simulink model "two_axes_motor_control"  (R2018a)
settings: Solver=VariableStepAuto  StartTime=0.0  StopTime=2700  RelTol=1e-3
undefined symbols (not defined in the file): b, J, Km, La, max_current, max_speed, Ra
libraries: simulink x6
settings Model: Creator=Ivonne  LastModifiedBy=Ivonne

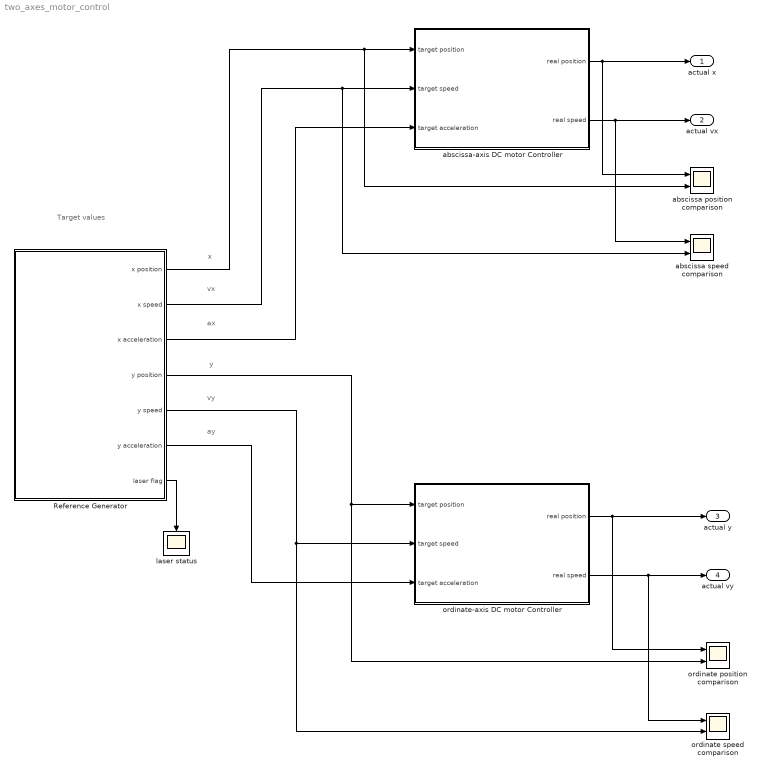
== system two_axes_motor_control ==
  note: x
  note: Target values
  note: vx
  note: ax
  note: y
  note: vy
  note: ay
  "Reference Generator " : Subsystem
  abscissa position comparison : Scope  NumInputPorts=2
  abscissa speed comparison : Scope  NumInputPorts=2
  abscissa-axis DC motor Controller : Subsystem
  laser status : Scope
  ordinate position comparison : Scope  NumInputPorts=2
  ordinate speed comparison : Scope  NumInputPorts=2
  ordinate-axis DC motor Controller : Subsystem
  actual x : Outport
  actual vx : Outport  Port=2
  actual y : Outport  Port=3
  actual vy : Outport  Port=4
  wires:
  "Reference Generator "/1("x position ") -> abscissa position comparison/2, abscissa-axis DC motor Controller/1(target position)
  "Reference Generator "/3("x acceleration ") -> abscissa-axis DC motor Controller/3(target acceleration)
  "Reference Generator "/2("x speed ") -> abscissa speed comparison/2, abscissa-axis DC motor Controller/2(target speed)
  "Reference Generator "/7("laser flag ") -> laser status/1
  abscissa-axis DC motor Controller/1(real position) -> abscissa position comparison/1, actual x/1
  abscissa-axis DC motor Controller/2(real speed) -> abscissa speed comparison/1, actual vx/1
  "Reference Generator "/4("y position ") -> ordinate position comparison/2, ordinate-axis DC motor Controller/1(target position)
  ordinate-axis DC motor Controller/1(real position) -> actual y/1, ordinate position comparison/1
  "Reference Generator "/6("y acceleration ") -> ordinate-axis DC motor Controller/3(target acceleration)
  "Reference Generator "/5("y speed ") -> ordinate-axis DC motor Controller/2(target speed), ordinate speed comparison/2
  ordinate-axis DC motor Controller/2(real speed) -> ordinate speed comparison/1, actual vy/1

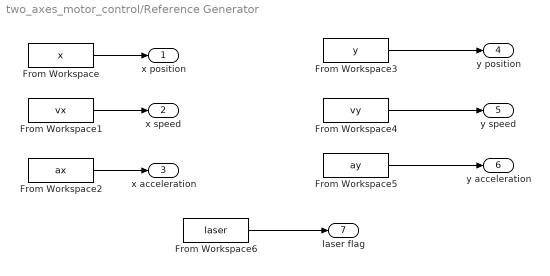
== system two_axes_motor_control/Reference Generator  ==
  From Workspace : FromWorkspace  VariableName=x  SampleTime=0  OutputAfterFinalValue=Holding final value
  From Workspace1 : FromWorkspace  VariableName=vx  SampleTime=0  OutputAfterFinalValue=Holding final value
  From Workspace2 : FromWorkspace  VariableName=ax  SampleTime=0  OutputAfterFinalValue=Holding final value
  From Workspace3 : FromWorkspace  VariableName=y  SampleTime=0  OutputAfterFinalValue=Holding final value
  From Workspace4 : FromWorkspace  VariableName=vy  SampleTime=0  OutputAfterFinalValue=Holding final value
  From Workspace5 : FromWorkspace  VariableName=ay  SampleTime=0  OutputAfterFinalValue=Holding final value
  From Workspace6 : FromWorkspace  VariableName=laser  SampleTime=0  Interpolate=off  OutputAfterFinalValue=Setting to zero
  "x position " : Outport
  "x speed " : Outport  Port=2
  "x acceleration " : Outport  Port=3
  "y position " : Outport  Port=4
  "y speed " : Outport  Port=5
  "y acceleration " : Outport  Port=6
  "laser flag " : Outport  Port=7
  wires:
  From Workspace/1 -> "x position "/1
  From Workspace5/1 -> "y acceleration "/1
  From Workspace3/1 -> "y position "/1
  From Workspace6/1 -> "laser flag "/1
  From Workspace2/1 -> "x acceleration "/1
  From Workspace4/1 -> "y speed "/1
  From Workspace1/1 -> "x speed "/1

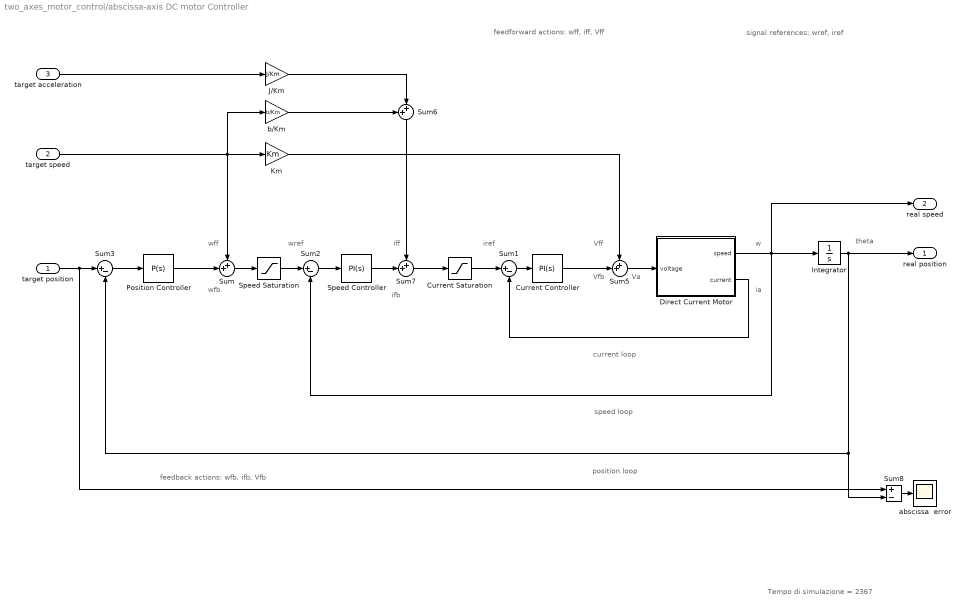
== system two_axes_motor_control/abscissa-axis DC motor Controller ==
  note: Tempo di simulazione = 2367
  note: ia
  note: theta
  note: w
  note: Va
  note: Vfb
  note: Vff
  note: signal references: wref, iref
  note: iref
  note: ifb
  note: iff
  note: wref
  note: wfb
  note: wff
  note: feedforward actions: wff, iff, Vff
  note: position loop
  note: speed loop
  note: current loop
  note: feedback actions: wfb, ifb, Vfb
  target position : Inport
  target speed : Inport  Port=2
  target acceleration : Inport  Port=3
  Current Controller : simulink/Continuous/PID Controller  Controller=PI  TimeDomain=Continuous-time  SampleTime=-1  IntegratorMethod=Forward Euler  FilterMethod=Forward Euler  Form=Parallel  UseFilter=on  ControllerParametersSource=internal  P=5000  I=10000  D=0  N=100  InitialConditionSource=internal  InitialConditionForIntegrator=0  InitialConditionForFilter=0  ExternalReset=none  LimitOutput=off  UpperSaturationLimit=inf  LowerSaturationLimit=-inf  LinearizeAsGain=on  AntiWindupMode=none  Kb=1  TrackingMode=off  Kt=1  PParamMin=[]  PParamMax=[]  IParamMin=[]  IParamMax=[]  DParamMin=[]  DParamMax=[]  NParamMin=[]  NParamMax=[]  KbParamMin=[]  KbParamMax=[]  KtParamMin=[]  KtParamMax=[]  POutMin=[]  POutMax=[]  IOutMin=[]  IOutMax=[]  DOutMin=[]  DOutMax=[]  NOutMin=[]  NOutMax=[]  KbOutMin=[]  KbOutMax=[]  KtOutMin=[]  KtOutMax=[]  IntegratorOutMin=[]  IntegratorOutMax=[]  FilterOutMin=[]  FilterOutMax=[]  SumOutMin=[]  SumOutMax=[]  SumI1OutMin=[]  SumI1OutMax=[]  SumI2OutMin=[]  SumI2OutMax=[]  SumI3OutMin=[]  SumI3OutMax=[]  SumDOutMin=[]  SumDOutMax=[]  SaturationOutMin=[]  SaturationOutMax=[]  IntegratorContinuousStateAttributes=''  IntegratorStateMustResolveToSignalObject=off  IntegratorRTWStateStorageClass=Auto  FilterContinuousStateAttributes=''  FilterStateMustResolveToSignalObject=off  FilterRTWStateStorageClass=Auto  DifferentiatorICPrevScaledInput=0  DifferentiatorOutMin=[]  DifferentiatorOutMax=[]  FilterDiffOutCoefMin=[]  FilterDiffOutCoefMax=[]  SumDenOutMin=[]  SumDenOutMax=[]  SumNumOutMin=[]  SumNumOutMax=[]  ReciprocalOutMin=[]  ReciprocalOutMax=[]  DivideOutMin=[]  DivideOutMax=[]  TunerSelectOption=Frequency Response Based
  Current Saturation : Saturate  UpperLimit=max_current  LowerLimit=-max_current
  Direct Current Motor : Subsystem
  Integrator : Integrator
  J/Km : Gain  Gain=J/Km
  Km : Gain  Gain=Km
  Position Controller : simulink/Continuous/PID Controller  Controller=P  TimeDomain=Continuous-time  SampleTime=-1  IntegratorMethod=Forward Euler  FilterMethod=Forward Euler  Form=Parallel  UseFilter=on  ControllerParametersSource=internal  P=10  I=1  D=0  N=100  InitialConditionSource=internal  InitialConditionForIntegrator=0  InitialConditionForFilter=0  ExternalReset=none  LimitOutput=off  UpperSaturationLimit=inf  LowerSaturationLimit=-inf  LinearizeAsGain=on  AntiWindupMode=none  Kb=1  TrackingMode=off  Kt=1  PParamMin=[]  PParamMax=[]  IParamMin=[]  IParamMax=[]  DParamMin=[]  DParamMax=[]  NParamMin=[]  NParamMax=[]  KbParamMin=[]  KbParamMax=[]  KtParamMin=[]  KtParamMax=[]  POutMin=[]  POutMax=[]  IOutMin=[]  IOutMax=[]  DOutMin=[]  DOutMax=[]  NOutMin=[]  NOutMax=[]  KbOutMin=[]  KbOutMax=[]  KtOutMin=[]  KtOutMax=[]  IntegratorOutMin=[]  IntegratorOutMax=[]  FilterOutMin=[]  FilterOutMax=[]  SumOutMin=[]  SumOutMax=[]  SumI1OutMin=[]  SumI1OutMax=[]  SumI2OutMin=[]  SumI2OutMax=[]  SumI3OutMin=[]  SumI3OutMax=[]  SumDOutMin=[]  SumDOutMax=[]  SaturationOutMin=[]  SaturationOutMax=[]  IntegratorContinuousStateAttributes=''  IntegratorStateMustResolveToSignalObject=off  IntegratorRTWStateStorageClass=Auto  FilterContinuousStateAttributes=''  FilterStateMustResolveToSignalObject=off  FilterRTWStateStorageClass=Auto  DifferentiatorICPrevScaledInput=0  DifferentiatorOutMin=[]  DifferentiatorOutMax=[]  FilterDiffOutCoefMin=[]  FilterDiffOutCoefMax=[]  SumDenOutMin=[]  SumDenOutMax=[]  SumNumOutMin=[]  SumNumOutMax=[]  ReciprocalOutMin=[]  ReciprocalOutMax=[]  DivideOutMin=[]  DivideOutMax=[]  TunerSelectOption=Frequency Response Based
  Speed Controller : simulink/Continuous/PID Controller  Controller=PI  TimeDomain=Continuous-time  SampleTime=-1  IntegratorMethod=Forward Euler  FilterMethod=Forward Euler  Form=Parallel  UseFilter=on  ControllerParametersSource=internal  P=200  I=400  D=0  N=100  InitialConditionSource=internal  InitialConditionForIntegrator=0  InitialConditionForFilter=0  ExternalReset=none  LimitOutput=off  UpperSaturationLimit=inf  LowerSaturationLimit=-inf  LinearizeAsGain=on  AntiWindupMode=none  Kb=1  TrackingMode=off  Kt=1  PParamMin=[]  PParamMax=[]  IParamMin=[]  IParamMax=[]  DParamMin=[]  DParamMax=[]  NParamMin=[]  NParamMax=[]  KbParamMin=[]  KbParamMax=[]  KtParamMin=[]  KtParamMax=[]  POutMin=[]  POutMax=[]  IOutMin=[]  IOutMax=[]  DOutMin=[]  DOutMax=[]  NOutMin=[]  NOutMax=[]  KbOutMin=[]  KbOutMax=[]  KtOutMin=[]  KtOutMax=[]  IntegratorOutMin=[]  IntegratorOutMax=[]  FilterOutMin=[]  FilterOutMax=[]  SumOutMin=[]  SumOutMax=[]  SumI1OutMin=[]  SumI1OutMax=[]  SumI2OutMin=[]  SumI2OutMax=[]  SumI3OutMin=[]  SumI3OutMax=[]  SumDOutMin=[]  SumDOutMax=[]  SaturationOutMin=[]  SaturationOutMax=[]  IntegratorContinuousStateAttributes=''  IntegratorStateMustResolveToSignalObject=off  IntegratorRTWStateStorageClass=Auto  FilterContinuousStateAttributes=''  FilterStateMustResolveToSignalObject=off  FilterRTWStateStorageClass=Auto  DifferentiatorICPrevScaledInput=0  DifferentiatorOutMin=[]  DifferentiatorOutMax=[]  FilterDiffOutCoefMin=[]  FilterDiffOutCoefMax=[]  SumDenOutMin=[]  SumDenOutMax=[]  SumNumOutMin=[]  SumNumOutMax=[]  ReciprocalOutMin=[]  ReciprocalOutMax=[]  DivideOutMin=[]  DivideOutMax=[]  TunerSelectOption=Frequency Response Based
  Speed Saturation : Saturate  UpperLimit=max_speed  LowerLimit=-max_speed
  Sum{,5..7} (4 alike) : Sum  Inputs=++|
  Sum1 : Sum  Inputs=|+-
  Sum2 : Sum  Inputs=|+-
  Sum3 : Sum  Inputs=|+-
  Sum8 : Sum  Inputs=+-
  abscissa  error : Scope
  b/Km : Gain  Gain=b/Km
  real position : Outport
  real speed : Outport  Port=2
  wires:
  Sum6/1 -> Sum7/1
  Direct Current Motor/1(speed) -> Sum2/2, Integrator/1, real speed/1
  Current Saturation/1 -> Sum1/1
  target speed/1 -> b/Km/1, Km/1, Sum/1
  Sum2/1 -> Speed Controller/1
  Speed Saturation/1 -> Sum2/1
  target position/1 -> Sum8/1, Sum3/1
  Current Controller/1 -> Sum5/2
  Sum5/1 -> Direct Current Motor/1(voltage)
  b/Km/1 -> Sum6/1
  Speed Controller/1 -> Sum7/2
  Position Controller/1 -> Sum/2
  Integrator/1 -> Sum8/2, Sum3/2, real position/1
  target acceleration/1 -> J/Km/1
  Direct Current Motor/2(current) -> Sum1/2
  Sum3/1 -> Position Controller/1
  Sum/1 -> Speed Saturation/1
  J/Km/1 -> Sum6/2
  Km/1 -> Sum5/1
  Sum1/1 -> Current Controller/1
  Sum7/1 -> Current Saturation/1
  Sum8/1 -> abscissa  error/1

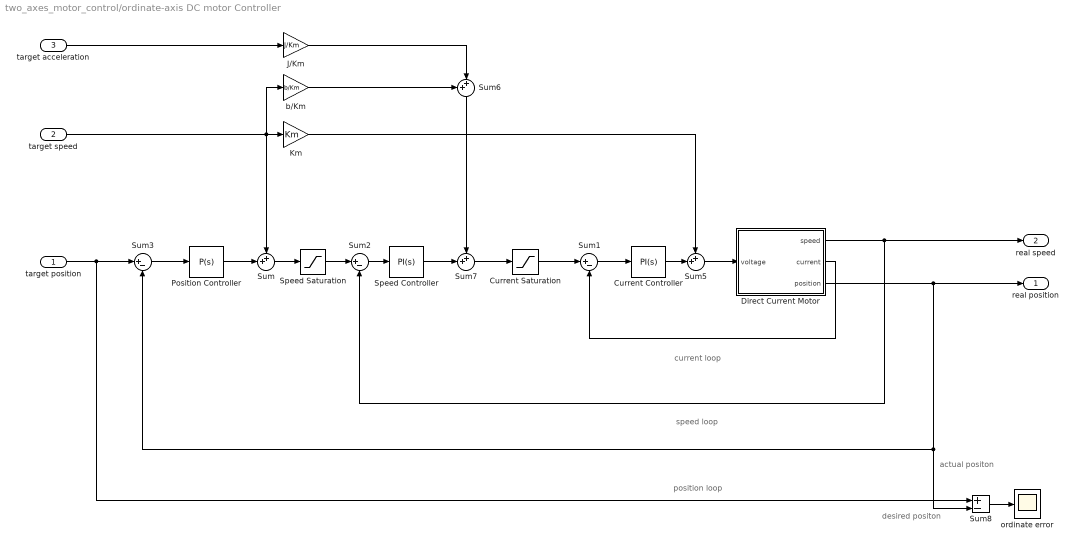
== system two_axes_motor_control/ordinate-axis DC motor Controller ==
  note: desired
      | positon
  note: position loop
  note: speed loop
  note: current loop
  note: actual
      | positon
  target position : Inport
  target speed : Inport  Port=2
  target acceleration : Inport  Port=3
  Current Controller : simulink/Continuous/PID Controller  Controller=PI  TimeDomain=Continuous-time  SampleTime=-1  IntegratorMethod=Forward Euler  FilterMethod=Forward Euler  Form=Parallel  UseFilter=on  ControllerParametersSource=internal  P=100  I=300  D=0  N=100  InitialConditionSource=internal  InitialConditionForIntegrator=0  InitialConditionForFilter=0  ExternalReset=none  LimitOutput=off  UpperSaturationLimit=inf  LowerSaturationLimit=-inf  LinearizeAsGain=on  AntiWindupMode=none  Kb=1  TrackingMode=off  Kt=1  PParamMin=[]  PParamMax=[]  IParamMin=[]  IParamMax=[]  DParamMin=[]  DParamMax=[]  NParamMin=[]  NParamMax=[]  KbParamMin=[]  KbParamMax=[]  KtParamMin=[]  KtParamMax=[]  POutMin=[]  POutMax=[]  IOutMin=[]  IOutMax=[]  DOutMin=[]  DOutMax=[]  NOutMin=[]  NOutMax=[]  KbOutMin=[]  KbOutMax=[]  KtOutMin=[]  KtOutMax=[]  IntegratorOutMin=[]  IntegratorOutMax=[]  FilterOutMin=[]  FilterOutMax=[]  SumOutMin=[]  SumOutMax=[]  SumI1OutMin=[]  SumI1OutMax=[]  SumI2OutMin=[]  SumI2OutMax=[]  SumI3OutMin=[]  SumI3OutMax=[]  SumDOutMin=[]  SumDOutMax=[]  SaturationOutMin=[]  SaturationOutMax=[]  IntegratorContinuousStateAttributes=''  IntegratorStateMustResolveToSignalObject=off  IntegratorRTWStateStorageClass=Auto  FilterContinuousStateAttributes=''  FilterStateMustResolveToSignalObject=off  FilterRTWStateStorageClass=Auto  DifferentiatorICPrevScaledInput=0  DifferentiatorOutMin=[]  DifferentiatorOutMax=[]  FilterDiffOutCoefMin=[]  FilterDiffOutCoefMax=[]  SumDenOutMin=[]  SumDenOutMax=[]  SumNumOutMin=[]  SumNumOutMax=[]  ReciprocalOutMin=[]  ReciprocalOutMax=[]  DivideOutMin=[]  DivideOutMax=[]  TunerSelectOption=Transfer Function Based (PID Tuner App)
  Current Saturation : Saturate  UpperLimit=max_current  LowerLimit=-max_current
  Direct Current Motor : Subsystem
  J/Km : Gain  Gain=J/Km
  Km : Gain  Gain=Km
  Position Controller : simulink/Continuous/PID Controller  Controller=P  TimeDomain=Continuous-time  SampleTime=-1  IntegratorMethod=Forward Euler  FilterMethod=Forward Euler  Form=Parallel  UseFilter=on  ControllerParametersSource=internal  P=1  I=1  D=0  N=100  InitialConditionSource=internal  InitialConditionForIntegrator=0  InitialConditionForFilter=0  ExternalReset=none  LimitOutput=off  UpperSaturationLimit=inf  LowerSaturationLimit=-inf  LinearizeAsGain=on  AntiWindupMode=none  Kb=1  TrackingMode=off  Kt=1  PParamMin=[]  PParamMax=[]  IParamMin=[]  IParamMax=[]  DParamMin=[]  DParamMax=[]  NParamMin=[]  NParamMax=[]  KbParamMin=[]  KbParamMax=[]  KtParamMin=[]  KtParamMax=[]  POutMin=[]  POutMax=[]  IOutMin=[]  IOutMax=[]  DOutMin=[]  DOutMax=[]  NOutMin=[]  NOutMax=[]  KbOutMin=[]  KbOutMax=[]  KtOutMin=[]  KtOutMax=[]  IntegratorOutMin=[]  IntegratorOutMax=[]  FilterOutMin=[]  FilterOutMax=[]  SumOutMin=[]  SumOutMax=[]  SumI1OutMin=[]  SumI1OutMax=[]  SumI2OutMin=[]  SumI2OutMax=[]  SumI3OutMin=[]  SumI3OutMax=[]  SumDOutMin=[]  SumDOutMax=[]  SaturationOutMin=[]  SaturationOutMax=[]  IntegratorContinuousStateAttributes=''  IntegratorStateMustResolveToSignalObject=off  IntegratorRTWStateStorageClass=Auto  FilterContinuousStateAttributes=''  FilterStateMustResolveToSignalObject=off  FilterRTWStateStorageClass=Auto  DifferentiatorICPrevScaledInput=0  DifferentiatorOutMin=[]  DifferentiatorOutMax=[]  FilterDiffOutCoefMin=[]  FilterDiffOutCoefMax=[]  SumDenOutMin=[]  SumDenOutMax=[]  SumNumOutMin=[]  SumNumOutMax=[]  ReciprocalOutMin=[]  ReciprocalOutMax=[]  DivideOutMin=[]  DivideOutMax=[]  TunerSelectOption=Transfer Function Based (PID Tuner App)
  Speed Controller : simulink/Continuous/PID Controller  Controller=PI  TimeDomain=Continuous-time  SampleTime=-1  IntegratorMethod=Forward Euler  FilterMethod=Forward Euler  Form=Parallel  UseFilter=on  ControllerParametersSource=internal  P=10  I=30  D=0  N=100  InitialConditionSource=internal  InitialConditionForIntegrator=0  InitialConditionForFilter=0  ExternalReset=none  LimitOutput=off  UpperSaturationLimit=inf  LowerSaturationLimit=-inf  LinearizeAsGain=on  AntiWindupMode=none  Kb=1  TrackingMode=off  Kt=1  PParamMin=[]  PParamMax=[]  IParamMin=[]  IParamMax=[]  DParamMin=[]  DParamMax=[]  NParamMin=[]  NParamMax=[]  KbParamMin=[]  KbParamMax=[]  KtParamMin=[]  KtParamMax=[]  POutMin=[]  POutMax=[]  IOutMin=[]  IOutMax=[]  DOutMin=[]  DOutMax=[]  NOutMin=[]  NOutMax=[]  KbOutMin=[]  KbOutMax=[]  KtOutMin=[]  KtOutMax=[]  IntegratorOutMin=[]  IntegratorOutMax=[]  FilterOutMin=[]  FilterOutMax=[]  SumOutMin=[]  SumOutMax=[]  SumI1OutMin=[]  SumI1OutMax=[]  SumI2OutMin=[]  SumI2OutMax=[]  SumI3OutMin=[]  SumI3OutMax=[]  SumDOutMin=[]  SumDOutMax=[]  SaturationOutMin=[]  SaturationOutMax=[]  IntegratorContinuousStateAttributes=''  IntegratorStateMustResolveToSignalObject=off  IntegratorRTWStateStorageClass=Auto  FilterContinuousStateAttributes=''  FilterStateMustResolveToSignalObject=off  FilterRTWStateStorageClass=Auto  DifferentiatorICPrevScaledInput=0  DifferentiatorOutMin=[]  DifferentiatorOutMax=[]  FilterDiffOutCoefMin=[]  FilterDiffOutCoefMax=[]  SumDenOutMin=[]  SumDenOutMax=[]  SumNumOutMin=[]  SumNumOutMax=[]  ReciprocalOutMin=[]  ReciprocalOutMax=[]  DivideOutMin=[]  DivideOutMax=[]  TunerSelectOption=Transfer Function Based (PID Tuner App)
  Speed Saturation : Saturate  UpperLimit=max_speed  LowerLimit=-max_speed
  Sum{,5..7} (4 alike) : Sum  Inputs=++|
  Sum1 : Sum  Inputs=|+-
  Sum2 : Sum  Inputs=|+-
  Sum3 : Sum  Inputs=|+-
  Sum8 : Sum  Inputs=+-
  b/Km : Gain  Gain=b/Km
  ordinate error : Scope
  real position : Outport
  real speed : Outport  Port=2
  wires:
  Sum6/1 -> Sum7/1
  Direct Current Motor/1(speed) -> Sum2/2, real speed/1
  Current Saturation/1 -> Sum1/1
  target speed/1 -> b/Km/1, Km/1, Sum/1
  Sum2/1 -> Speed Controller/1
  Speed Saturation/1 -> Sum2/1
  target position/1 -> Sum8/1, Sum3/1
  Current Controller/1 -> Sum5/2
  Sum5/1 -> Direct Current Motor/1(voltage)
  b/Km/1 -> Sum6/1
  Speed Controller/1 -> Sum7/2
  Position Controller/1 -> Sum/2
  Direct Current Motor/3(position) -> real position/1, Sum8/2, Sum3/2
  target acceleration/1 -> J/Km/1
  Direct Current Motor/2(current) -> Sum1/2
  Sum3/1 -> Position Controller/1
  Sum/1 -> Speed Saturation/1
  J/Km/1 -> Sum6/2
  Km/1 -> Sum5/1
  Sum1/1 -> Current Controller/1
  Sum7/1 -> Current Saturation/1
  Sum8/1 -> ordinate error/1

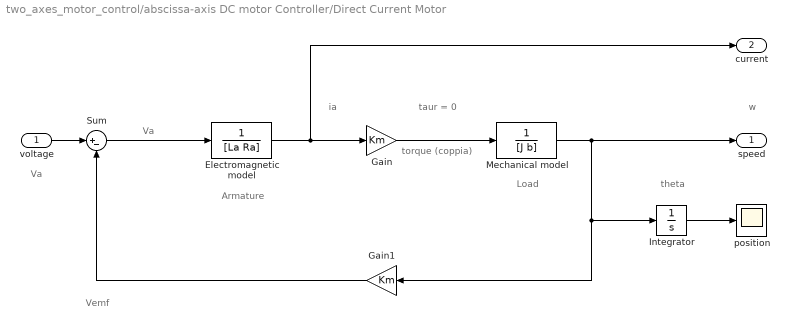
== system two_axes_motor_control/abscissa-axis DC motor Controller/Direct Current Motor ==
  note: Vemf
  note: Va
  note: Load
  note: Armature
  note: theta
  note: w
  note: ia
  note: taur = 0
  note: Va
  note: torque (coppia)
  voltage : Inport
  Electromagnetic model : TransferFcn  Denominator=[La Ra]
  Gain : Gain  Gain=Km
  Gain1 : Gain  Gain=Km
  Integrator : Integrator
  Mechanical model : TransferFcn  Denominator=[J b]
  Sum : Sum  Inputs=|+-
  position : Scope
  speed : Outport
  current : Outport  Port=2
  wires:
  Gain/1 -> Mechanical model/1
  Mechanical model/1 -> Gain1/1, Integrator/1, speed/1
  Electromagnetic model/1 -> current/1, Gain/1
  Sum/1 -> Electromagnetic model/1
  voltage/1 -> Sum/1
  Gain1/1 -> Sum/2
  Integrator/1 -> position/1

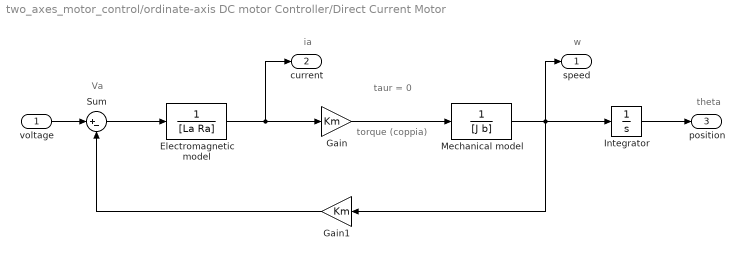
== system two_axes_motor_control/ordinate-axis DC motor Controller/Direct Current Motor ==
  note: theta
  note: w
  note: ia
  note: taur = 0
  note: Va
  note: torque (coppia)
  voltage : Inport
  Electromagnetic model : TransferFcn  Denominator=[La Ra]
  Gain : Gain  Gain=Km
  Gain1 : Gain  Gain=Km
  Integrator : Integrator
  Mechanical model : TransferFcn  Denominator=[J b]
  Sum : Sum  Inputs=|+-
  speed : Outport
  current : Outport  Port=2
  position : Outport  Port=3
  wires:
  Gain/1 -> Mechanical model/1
  Mechanical model/1 -> Gain1/1, speed/1, Integrator/1
  Electromagnetic model/1 -> current/1, Gain/1
  Integrator/1 -> position/1
  voltage/1 -> Sum/1
  Sum/1 -> Electromagnetic model/1
  Gain1/1 -> Sum/2
